simulink model "bu_abslut125_romvect_float"  (R2021b)
settings: Solver=VariableStepAuto  StartTime=0.0  StopTime=350  RelTol=1e-3
undefined symbols (not defined in the file or in its folder): figd2104, xcu250
libraries: hdlBasic x1696, vmcUtilities x1
(part 1 of 8)
settings Model: Creator=shu_abe  LastModifiedBy=shu_abe

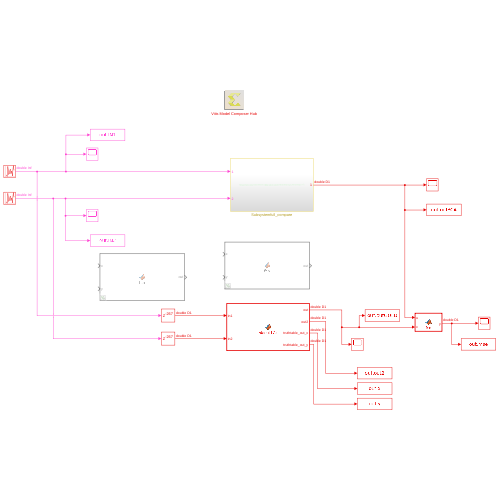
[thumbnail: Simulink's stored preview of the top-level diagram]
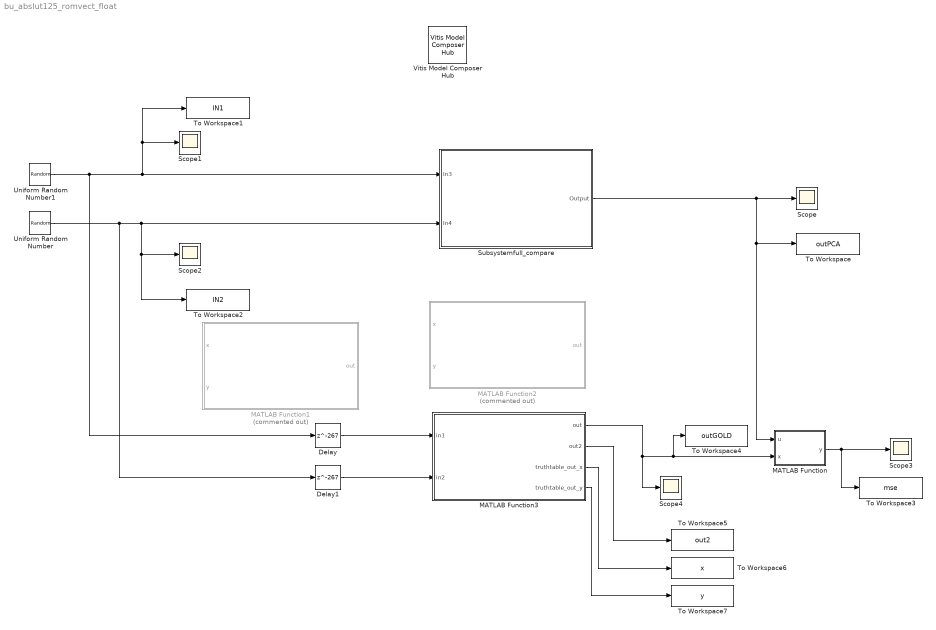
== system bu_abslut125_romvect_float ==
  Delay : Delay  DelayLength=267
  Delay1 : Delay  DelayLength=267
  MATLAB Function : MATLAB Function  TreatAsAtomicUnit=on
  MATLAB Function1 : MATLAB Function  Commented=on  TreatAsAtomicUnit=on
  MATLAB Function2 : MATLAB Function  Commented=on  TreatAsAtomicUnit=on
  MATLAB Function3 : MATLAB Function  TreatAsAtomicUnit=on
  Scope{,1..4} (5 alike) : Scope
  Subsystemfull_compare : Subsystem
  To Workspace : ToWorkspace  VariableName=outPCA  SaveFormat=Structure With Time  SampleTime=1
  To Workspace1 : ToWorkspace  VariableName=IN1  SaveFormat=Structure With Time  SampleTime=-1
  To Workspace2 : ToWorkspace  VariableName=IN2  SaveFormat=Structure With Time  SampleTime=-1
  To Workspace3 : ToWorkspace  VariableName=mse  SaveFormat=Structure With Time  SampleTime=1
  To Workspace4 : ToWorkspace  VariableName=outGOLD  SaveFormat=Structure With Time  SampleTime=1
  To Workspace5 : ToWorkspace  VariableName=out2  SaveFormat=Structure With Time  SampleTime=1
  To Workspace6 : ToWorkspace  VariableName=x  SaveFormat=Structure With Time  SampleTime=1
  To Workspace7 : ToWorkspace  VariableName=y  SaveFormat=Structure With Time  SampleTime=1
  Uniform Random Number : UniformRandomNumber  Minimum=0  SampleTime=1
  Uniform Random Number1 : UniformRandomNumber  Minimum=0  Seed=1  SampleTime=1
  Vitis Model Composer Hub : vmcUtilities/Vitis Model Composer Hub  Tag=genX  CodeGeneration=off  SubsystemName=<enter or select subsystem name>  TargetDirectory=./code  ExportType=HLS C++ code  IpVendor=xilinx.com  IpLibrary=hls  IpVersion=1.0  IpHWLanguage=Verilog  AieCompilerOptions={}  CreateTestbench=off  TestbenchStackSize=10  RunAieSim=off  AieSimTimeout=50000  RunAieSimProfiling=off  LaunchVitisAnalyzer=off  PlotOutput=off  RunX86Sim=off  X86SimTimeout=10  GenHwImage=off  PlatformType=Not Specified  HwSystemType=Baremetal  HwValidationTarget=hw  ProjDevice=Alveo U250 Data Center Accelerator Card (xcu250-figd2104-2L-e)  ProjDevicePart=xcu250-figd2104-2L-e  SamplePeriod=-1  ClockFrequency=200  DataPathParallelism=1  xilinxfamily=virtexuplus  part=xcu250  speed=-2L-e  package=figd2104  directory=./cordic_nopipe_08  testbench=on  incr_netlist=off  synthesis_tool=Vivado  clock_wrapper=Clock Enables  dbl_ovrd=According to Block Masks  dcm_input_clock_period=10  sysclk_period=10  simulink_period=1  eval_field=0
  wires:
  MATLAB Function/1(y) -> To Workspace3/1, Scope3/1
  Subsystemfull_compare/1(Output) -> Scope/1, MATLAB Function/1(u), To Workspace/1
  Uniform Random Number1/1 -> Subsystemfull_compare/1(In3), To Workspace1/1, Scope1/1, Delay/1
  Uniform Random Number/1 -> Subsystemfull_compare/2(In4), To Workspace2/1, Scope2/1, Delay1/1
  MATLAB Function3/1(out) -> Scope4/1, To Workspace4/1, MATLAB Function/2(x)
  Delay/1 -> MATLAB Function3/1(in1)
  Delay1/1 -> MATLAB Function3/2(in2)
  MATLAB Function3/2(out2) -> To Workspace5/1
  MATLAB Function3/3(truthtable_out_x) -> To Workspace6/1
  MATLAB Function3/4(truthtable_out_y) -> To Workspace7/1
